simulink model "Dyn_6DoF_v2_0_r2019b"  (R2022a)
settings: Solver=ode4  StartTime=0.0  StopTime=simInit.TSIM  FixedStep=simInit.dt  MaxStep=simInit.dt  RelTol=1e-3
InitFcn:
  | close all
undefined symbols (not defined in the file): act, constr, DE2019, DiscIntNeverNeededParam, ENVMT, omega_rate_max, params, simInit
libraries: simulink x14, simulink_extras x3
(part 3 of 3)

== matlab function Dyn_6DoF_v2_0_r2019b/AirborneSystem/ForcesAndTorques/aerodynamic forces FSI/Rudder Aero/Rudder_aero ==
  data: input input double; out output double size=[6,1]; DE2019 parameter; ENVMT parameter
% Copyright 2021 Delft University of Technology
%
% Licensed under the Apache License, Version 2.0 (the "License");
% you may not use this file except in compliance with the License.
% You may obtain a copy of the License at
%
%      http://www.apache.org/licenses/LICENSE-2.0
%
% Unless required by applicable law or agreed to in writing, software
% distributed under the License is distributed on an "AS IS" BASIS,
% WITHOUT WARRANTIES OR CONDITIONS OF ANY KIND, either express or implied.
% See the License for the specific language governing permissions and
% limitations under the License.

function out = simpleAero(input, DE2019, ENVMT)
%simpleAero - Rudder simple aero calculation
%
% Inputs:
%    input  - airspeed, AoA, sideslip, CL and CD
%    DE2019 - Aircraft parameters
%    ENVMT  - Environment characteristics
%
% Outputs:
%    out    - 3D forces and moments generated by the rudder
%
%
% Author: Sebastian Rapp, Ph.D., Revised by: Dylan Eijkelhof, M.Sc.
% Delft University of Technology
% email address: d.eijkelhof@tudelft.nl
% December 2019; Last revision: 19-March-2021

%-------------	BEGIN CODE	--------------
    V = input(1);
    alpha = input(2);
    beta = input(3);

    q = 0.5*ENVMT.rhos*V^2;
   
    F_L_vs = 2*input(4)*q*DE2019.S_vs;
    F_D_vs = -2*input(5)*q*DE2019.S_vs;

    F_x_s = F_D_vs*cos(alpha)*cos(beta);
    F_y_s = -F_L_vs*cos(beta);
    F_z_s = 0;

    M_x_s = F_L_vs*(DE2019.b_vs*0.5);
    M_y_s = 0;
    M_z_s = F_L_vs*(DE2019.x_vs+DE2019.c_vs*0.25);

    out = [F_x_s, F_y_s, F_z_s, M_x_s, M_y_s, M_z_s]';
%-------------	END CODE	--------------  
end

== matlab function Dyn_6DoF_v2_0_r2019b/RequirementModelsAndLogging/Power_convergence/MATLAB Function ==
  data: flag output; m_new output; p_sum output; cnt output; flag input; m_old input; p_sum input; cnt input; u input; flightMode input; e_new output; e_old input; cnt_max_mat input; cnt_max_mat output; cycles_cnt input; cycles_cnt output
% Copyright 2021 Delft University of Technology
%
% Licensed under the Apache License, Version 2.0 (the "License");
% you may not use this file except in compliance with the License.
% You may obtain a copy of the License at
%
%      http://www.apache.org/licenses/LICENSE-2.0
%
% Unless required by applicable law or agreed to in writing, software
% distributed under the License is distributed on an "AS IS" BASIS,
% WITHOUT WARRANTIES OR CONDITIONS OF ANY KIND, either express or implied.
% See the License for the specific language governing permissions and
% limitations under the License.

function [flag, m_new, p_sum, cnt, e_new, cnt_max_mat,cycles_cnt] = fcn(flag, m_old, p_sum, cnt, u, flightMode, e_old,cnt_max_mat,cycles_cnt)
% function [flag, m_new, p_sum, cnt, e_new, cnt_max_mat,cycles_cnt] = fcn(flag, m_old, p_sum, cnt, u, flightMode, e_old,cnt_max_mat,cycles_cnt, cnt_extra)
%y = [u;old(1:end-1)];
% if cnt > nmax
%     new_mean = mean(y);
%     cnt = 0;
% end
p_sum = p_sum + u;
cnt = cnt + 1;

if flightMode == 5 && flag
    cnt_max_mat = cnt; 
    m_new = p_sum/cnt;
    cnt  = 0;
    cycles_cnt = cycles_cnt + 1;
    p_sum = 0;
    flag = 0;
    e_new = abs( m_new - m_old );
elseif flightMode == 6
%     if cnt_extra == 0 || cycles_cnt == 0
%         cycles_cnt = cycles_cnt + 1;
%     end
    flag = 1;
    m_new = m_old;
    e_new = e_old;
else
    flag = 0;
    m_new = m_old;
    e_new = e_old;
end

% m_new = m_old + (u-old(nmax))/nmax;

== matlab function Dyn_6DoF_v2_0_r2019b/AirborneSystem/6DoFDynamics/Subsystem/Estimations ==
  data: Ft input; F_a_B input; F_p_B input; v_k_B input; v_w_W input; mu_k output; Va output; mu_a output; alpha output; beta output; chi_a_dot_real output; gamma_a_dot_real output; M_OB input; longlat input; EULER input; pathangles_a output; pathangles_k output; v_k_O output; pos_W output; pos_O output; ENVMT parameter; DE2019 parameter; v_k_W output; h_tau input
% Copyright 2021 Delft University of Technology
%
% Licensed under the Apache License, Version 2.0 (the "License");
% you may not use this file except in compliance with the License.
% You may obtain a copy of the License at
%
%      http://www.apache.org/licenses/LICENSE-2.0
%
% Unless required by applicable law or agreed to in writing, software
% distributed under the License is distributed on an "AS IS" BASIS,
% WITHOUT WARRANTIES OR CONDITIONS OF ANY KIND, either express or implied.
% See the License for the specific language governing permissions and
% limitations under the License.

function [mu_k,Va, mu_a, alpha, beta, chi_a_dot_real,gamma_a_dot_real, ...
    pathangles_a, pathangles_k, v_k_O, pos_W, pos_O, v_k_W] = ...
    fcn(Ft, F_a_B, F_p_B, v_k_B, v_w_W,M_OB,longlat,EULER,...
    ENVMT, DE2019, h_tau)
%fcn - 6DoF dynamics estimations
%
% Inputs:
%    Ft      - Tether force magnitude at the kite
%    F_a_B   - Aerodynamic forces acting on kite in body reference frames
%    F_p_B   - Propulsion and brake forces acting on kite in body reference
%              frames 
%    v_k_B   - Kinetic velocity in body reference frame
%    M_OB    - Rotation matrix from body to inertial reference frame
%    longlat - Longtitude, latitude
%    EULER   - Euler angles
%    ENVMT   - Environment characteristics
%    DE2019  - Aircraft parameters
%    h_tau   - Height in tau reference frame
%
% Outputs:
%    mu_k              - Kinetic roll angle
%    Va                - Airspeed (magnitude)
%    mu_a              - Aerodynamic roll angle
%    alpha             - Pitch angle
%    beta              - Sideslip(yaw) angle
%    chi_a_dot_real    - rate of change in aerodynamic course heading
%    gamma_a_dot_real  - rate of change in aerodynamic path angle
%    pathangles_a      - Aerodynamic course heading and path angle
%    pathangles_k      - Kinetic course heading and path angle
%    v_k_O             - Kinetic velocity in inertial reference frame
%    pos_W             - Kite position in wind reference frame
%    pos_O             - Kite position in inertial reference frame
%    v_k_W             - Kinetic velocity in wind reference frame
%
% Author: Sebastian Rapp, Ph.D., Revised by: Dylan Eijkelhof, M.Sc.
% Delft University of Technology
% email address: d.eijkelhof@tudelft.nl
% December 2019; Last revision: 19-March-2021

%-------------	BEGIN CODE	--------------
% Preallocate variables
mu_k             = 0;
Va               = 0;
mu_a             = 0;
alpha            = 0; 
beta             = 0;
chi_a_dot_real   = 0;
gamma_a_dot_real = 0;
pathangles_a     = zeros(2,1);
pathangles_k     = zeros(2,1); 
M_B2ABar         = zeros(3,3);

long = longlat(1);
lat  = longlat(2);

M_WO = [cos(ENVMT.windDirection_rad), sin(ENVMT.windDirection_rad), 0;
        sin(ENVMT.windDirection_rad), -cos(ENVMT.windDirection_rad), 0;
        0, 0, -1];
    
pos_W = [cos(long)*cos(lat);
         sin(long)*cos(lat);
         sin(lat)]*abs(h_tau);
    
pos_O = M_WO'*pos_W;   
v_k_O = M_OB*v_k_B;
v_k_W =  M_WO*v_k_O;

v_a_W = v_k_W - v_w_W;
Va = norm(v_a_W);

v_a_O = transformFromWtoO(ENVMT.windDirection_rad, v_a_W);
v_a_B = M_OB' * v_a_O;

chi_k        = atan2( v_k_O(2), v_k_O(1) );
gamma_k      = -asin( v_k_O(3)/norm(v_k_O) );
pathangles_k = [chi_k; gamma_k];

chi_a        = atan2( v_a_O(2), v_a_O(1) );
gamma_a      = -asin( v_a_O(3)/norm(v_a_O) );
pathangles_a = [chi_a; gamma_a];

% Estimation of aerodynamic angles 
alpha = atan2( v_a_B(3), v_a_B(1) );
beta  = asin( v_a_B(2)/norm(v_a_B) );
mu_a  = asin( max( min( (cos(EULER(2))*sin(EULER(1)))/(cos(gamma_a)*cos(beta)) ...
    + tan(gamma_a) * tan(beta), 1),-1) ); 

beta_k = atan2( v_k_B(2), norm(v_k_B) );
mu_k   = asin( max( min( (cos(EULER(2))*sin(EULER(1)))/(cos(gamma_k)*cos(beta_k)) ...
    + tan(gamma_k) * tan(beta_k), 1),-1) ); 

c_m = cos(mu_a);
s_m = sin(mu_a);

c_a = cos(alpha);
s_a = sin(alpha);

c_b = cos(beta);
s_b = sin(beta);

M_B2ABar(1,1) = c_a*c_b;
M_B2ABar(1,2) = s_b;
M_B2ABar(1,3) = s_a*c_b;
M_B2ABar(2,1) = -c_a*s_b*c_m+s_a*s_m;
M_B2ABar(2,2) = c_b*c_m;
M_B2ABar(2,3) = -s_a*s_b*c_m-s_m*c_a;
M_B2ABar(3,1) = -c_a*s_b*s_m-s_a*c_m;
M_B2ABar(3,2) = c_b*s_m;
M_B2ABar(3,3) = -s_a*s_b*s_m+c_a*c_m;

% Estimtion of chi_a_dot and gamma_a_dot
c_chia = cos(chi_a);
s_chia = sin(chi_a);

c_gama = cos(gamma_a);
s_gama = sin(gamma_a);

M_ABar2O = zeros(3,3);

M_ABar2O(1,1) = c_chia*c_gama;
M_ABar2O(2,1) = s_chia*c_gama;
M_ABar2O(3,1) = -s_gama;
M_ABar2O(1,2) = -s_chia;
M_ABar2O(2,2) = c_chia;
M_ABar2O(3,2) = 0;
M_ABar2O(1,3) = c_chia*s_gama;
M_ABar2O(2,3) = s_chia*s_gama;
M_ABar2O(3,3) = c_gama;


F_g_t_Abar  = M_ABar2O' * ( [0;0;DE2019.mass*ENVMT.g] -Ft*pos_O/norm(pos_O) );
F_ap_B      = M_B2ABar * (F_a_B+F_p_B);
f_y         = F_ap_B(2) + F_g_t_Abar(2); 
f_z         = F_ap_B(3) + F_g_t_Abar(3);

chi_a_dot_real   = 1/cos(gamma_a)/Va/DE2019.mass  * (f_y);
gamma_a_dot_real = -1/Va/DE2019.mass * (f_z);

%-------------	END CODE	--------------
end
